simulink model "seEstimatingAssemblyLineThroughput"  (R2020b)
settings: Solver=VariableStepAuto  StartTime=0.0  StopTime=86407  FixedStep=7  RelTol=1e-3
PostLoadFcn:
  | excelFile   = [matlabroot...
  |   '/examples/simevents/data/seEstimatingAssemblyLineThroughput.xlsx'];
  | 
  | schedule    = xlsread(excelFile, 'MfgSchedule');      % Part Scheduling information
  | optimes     = xlsread(excelFile, 'OperationTimes');  % Operation Times
  | parameters  = xlsread(excelFile, 'Parameters');      % Simulation Parameters
  | 
  | numMfgWorkers = parameters(1); 		 % number of workers in Manufacturing area
  | numInspectWorkers = parameters(2); 	 % number of workers in Inspection area
  | discard_rate = parameters(4)/100; 	                     % quality rejection rate
  | seed = 12345;                     	                     % random number seed
  | requirements = xlsread(excelFile, 'Requirements');
  | scheduleID = 4;                                                        % The column number to read from excel
undefined symbols (not defined in the file or in its folder): m, n, openFastenGate, openInspect1Gate, openInspect2Gate, openInspect3Gate, openMilling1Gate, openMilling2Gate
libraries: sldelib x4, bonsai_library x1
CloseFcn:
  | clear discard_rate excelFile logsout numInspectWorkers numMfgWorkers optimes parameters requirements schedule scheduleID seed;
settings Model: Creator=The MathWorks, Inc.  LastModifiedBy=jomcdowe
settings DataIOCC: SaveOutput=off  SaveTime=off  ReturnWorkspaceOutputs=off
settings DebuggingCC: ArithmeticOperatorsInVariantConditions=warning
settings SFSimCC: SimUseLocalCustomCode=off  CustomCodeUndefinedFunction=UseInterfaceOnly
settings RTWCC: RTWUseLocalCustomCode=off
settings CodeAppCC: StateflowObjectComments=on

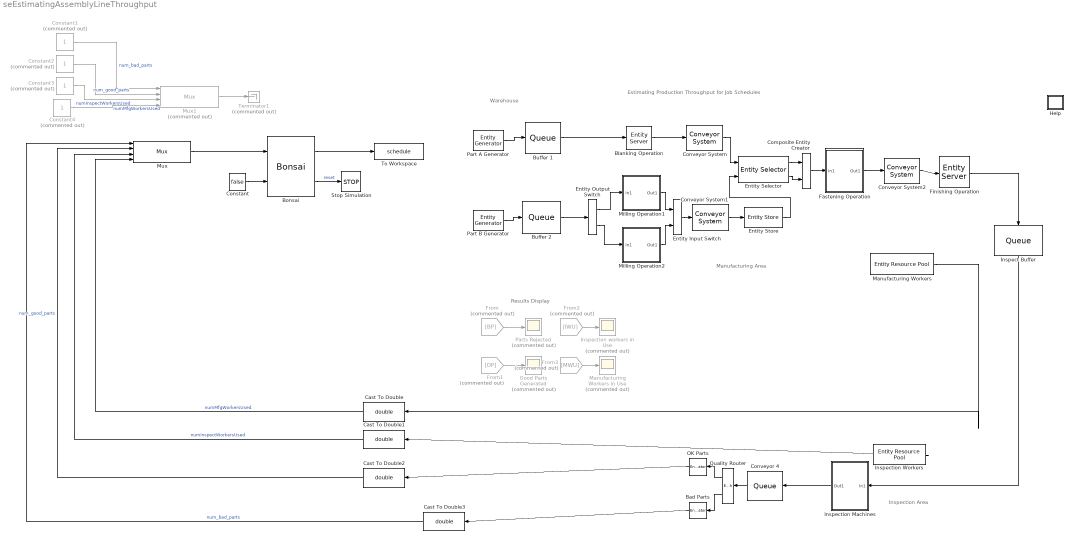
== system seEstimatingAssemblyLineThroughput ==
  note: Warehouse
  note: Results Display
  note: Manufacturing Area
  note: Estimating Production Throughput for Job Schedules
  note: Inspection Area
  Bad Parts : EntityTerminator  InputPortMessageModes=m  NumberEntitiesArrived=on
      settings: OutputPortMap=o0
  Blanking Operation : EntityServer  InputPortMessageModes=m  OutputPortMessageModes=m  Capacity=1  ServiceTimeSource=MATLAB action  ServiceTimeAction=|
      | % The times on the servers are going to vary
      | % as a normal dist, with std-dev of 'variation'.
      | 
      | persistent rngInit;
      | if isempty(rngInit)
      |     rng(seed);
      |     rngInit = true;
      | end
      | 
      | variation = parameters(5)/100;    % variation over nominal
      | nominalTime = optimes(entity.Variant, 2);
      | stdDev = nominalTime*variation;
      | 
      | % Pattern: Gaussian (normal) distribution
      | dt = nominalTime + stdDev * randn;
      mask Display: image([matlabroot,'/examples/simevents/data/SLDEBlanking.gif']);
  Bonsai : bonsai_library/Bonsai  sampleTime=[68400, 0]
      settings: SourceProductName=Bonsai Toolbox
  Buffer 1 : Queue  InputPortMessageModes=m  OutputPortMessageModes=m  Capacity=4
      mask Display: image([matlabroot,'/examples/simevents/data/SLDEPallet.png']);
  Buffer 2 : Queue  InputPortMessageModes=m  OutputPortMessageModes=m  Capacity=4
      mask Display: image([matlabroot,'/examples/simevents/data/SLDEPallet.png']);
  Cast To Double{,1..3} (4 alike) : DataTypeConversion  OutDataTypeStr=double
  Composite Entity Creator : CompositeEntityCreator  InputPortMessageModes=m,m  OutputPortMessageModes=m  EntityTypeName=Combined  InputEntityName=Part_A|Part_B
      settings: InputPortMap=u0,u1
  Constant : Constant  Value=false
  Constant{1..4} (4 alike) : Constant  Commented=on
  Conveyor 4 : Queue  InputPortMessageModes=m  OutputPortMessageModes=m  Capacity=2  EntryAction=|
      | % Set the percentage of parts
      | % that have to be discarded
      | % discard_rate = 0.05;
      | 
      | flip = rand();
      | if flip > discard_rate
      |     entity.Part_A.Rework = 1;    % rework not needed
      | else
      |     entity.Part_A.Rework = 2;    % rework needed
      | end
      mask Display: image([matlabroot,'/examples/simevents/data/SLDEFlatPallet.jpg']);
  Conveyor System : sldelib/Conveyor System  mConveyorLength=100  mConveyorSpeedSource=Dialog  mConveyorSpeed=20  mInitialConveyorSpeed=1000  mMinDisBetEntity=0  mEntityLengthSource=Dialog  mEntityLength=30  mEntityLengthAttrName=Length  mOutputBlockedOpt=Accumulate  mErrorUponFullOpt=off  mNumEntitiesDepOpt=off  mNumEntitiesInBlockOpt=off  mEntityPendingOpt=off  mNumExtractedFromBlockOpt=off  mConveyorSpeedOpt=off
      settings: SourceProductName=SimEvents
  Conveyor System1 : sldelib/Conveyor System  mConveyorLength=100  mConveyorSpeedSource=Dialog  mConveyorSpeed=20  mInitialConveyorSpeed=1000  mMinDisBetEntity=0  mEntityLengthSource=Dialog  mEntityLength=30  mEntityLengthAttrName=Length  mOutputBlockedOpt=Accumulate  mErrorUponFullOpt=off  mNumEntitiesDepOpt=off  mNumEntitiesInBlockOpt=off  mEntityPendingOpt=off  mNumExtractedFromBlockOpt=off  mConveyorSpeedOpt=off
      settings: SourceProductName=SimEvents
  Conveyor System2 : sldelib/Conveyor System  mConveyorLength=100  mConveyorSpeedSource=Dialog  mConveyorSpeed=20  mInitialConveyorSpeed=1000  mMinDisBetEntity=0  mEntityLengthSource=Dialog  mEntityLength=30  mEntityLengthAttrName=Length  mOutputBlockedOpt=Accumulate  mErrorUponFullOpt=off  mNumEntitiesDepOpt=off  mNumEntitiesInBlockOpt=off  mEntityPendingOpt=off  mNumExtractedFromBlockOpt=off  mConveyorSpeedOpt=off
      settings: SourceProductName=SimEvents
  Entity Input Switch : EntityInputSwitch  InputPortMessageModes=m,m  OutputPortMessageModes=m
  Entity Output Switch : EntityOutputSwitch  InputPortMessageModes=m  OutputPortMessageModes=m,m  SwitchAttributeName=Attribute1
  Entity Selector : sldelib/Entity Selector  mNumberOfStreams=1  mKeyEntityAttributeName='Variant'  mEntityAttributeName='VariantB'  mMatchingNumberSource=Dialog  mNumberOfMatches=1  mNumberOfMatchesAttribute=Name  mNumEntitiesDepOpt=off  mNumEntitiesInBlockOpt=off  mNumEntitiesExtractedOpt=off
      settings: SourceProductName=SimEvents
  Entity Store : EntityStore  InputPortMessageModes=m  OutputPortMessageModes=m  Capacity=4
      settings: OutputPortMap=o4
  Fastening Operation : Subsystem
      mask Display: image([matlabroot,'/examples/simevents/data/SLDEFasteningMachine.jpg']);
  Finishing Operation : EntityServer  InputPortMessageModes=m  OutputPortMessageModes=m  Capacity=1  ServiceTimeSource=MATLAB action  ServiceTimeAction=|
      | % The times on the servers are going to vary
      | % as a normal dist, with std-dev of 'variation'.
      | 
      | persistent rngInit;
      | if isempty(rngInit)
      |     rng(seed);
      |     rngInit = true;
      | end
      | 
      | variation = parameters(5)/100;    % variation over nominal
      | nominalTime = optimes(entity.Part_A.Variant, 6);
      | stdDev = nominalTime*variation;
      | 
      | % Pattern: Gaussian (normal) distribution
      | dt = nominalTime + stdDev * randn;
      mask Display: image([matlabroot,'/examples/simevents/data/SLDEFinishing.jpg']);
  From : From  Commented=on  GotoTag=BP
  From1 : From  Commented=on  GotoTag=OP
  From2 : From  Commented=on  GotoTag=IWU
  From3 : From  Commented=on  GotoTag=MWU
  Good Parts Generated : Scope  Commented=on
  Help : Subsystem
      settings: OpenFcn=showExample('simevents/EstimatingAssemblyLineThroughputExample');
      mask Display: disp('?')
  Inspect Buffer : Queue  InputPortMessageModes=m  OutputPortMessageModes=m  Capacity=4
      mask Display: image([matlabroot,'/examples/simevents/data/SLDEPallet.png']);
  Inspection Machines : Subsystem
      mask Display: image([matlabroot,'/examples/simevents/data/SLDEInspectMachine.png']);
  Inspection Workers : EntityResourcePool  ResourceName=InspectionWorkers  ResourceAmount=numInspectWorkers  AmountInUse=on
  Inspection workers in Use : Scope  Commented=on
  Manufacturing Workers : EntityResourcePool  ResourceName=MillingFasteningWorkers  ResourceAmount=numMfgWorkers  AmountInUse=on
  Manufacturing Workers in Use : Scope  Commented=on
  Milling Operation1 : Subsystem
      mask Display: image([matlabroot,'/examples/simevents/data/SLDEMillingMachine.jpg']);
  Milling Operation2 : Subsystem
      mask Display: image([matlabroot,'/examples/simevents/data/SLDEMillingMachine.jpg']);
  Mux : Mux
      settings: DisplayOption=signals
  Mux1 : Mux  Commented=on
      settings: DisplayOption=signals
  OK Parts : EntityTerminator  InputPortMessageModes=m  NumberEntitiesArrived=on
      settings: OutputPortMap=o0
  Part A Generator : EntityGenerator  OutputPortMessageModes=m  TimeSource=MATLAB action  IntergenerationTimeAction=|  GenerateAction=|  AttributeName=Rework|Variant  AttributeInitialValue=1|1  EntityType=Structured  EntityTypeName=Part_A
      | persistent idx;
      | if isempty(idx)
      |     idx = 1;
      | end
      | 
      | % Set the Inter Generation Time (IGT)
      | dt = schedule(idx, 1);
      | if idx < length(schedule(:, 1))
      |     idx = idx + 1;
      | else
      |     idx = 1;    % go back to first part
      | end
      | persistent idx;
      | if isempty(idx)
      |     idx = 1;
      | end
      | 
      | % Set the variant
      | entity.Variant = schedule(idx, scheduleID);
      | 
      | % Book-keeping work
      | if idx < length(schedule(:, 1))
      |     idx = idx + 1;
      | else
      |     idx = 1;    % go back to first part
      | end
  Part B Generator : EntityGenerator  OutputPortMessageModes=m  TimeSource=MATLAB action  IntergenerationTimeAction=|  GenerateAction=|  AttributeName=VariantB  EntityType=Structured  EntityTypeName=Part_B
      | persistent idx;
      | if isempty(idx)
      |     idx = 1;
      | end
      | 
      | % Set the Inter Generation Time (IGT)
      | dt = schedule(idx, 1);
      | if idx < length(schedule(:, 1))
      |     idx = idx + 1;
      | else
      |     idx = 1;    % go back to first part
      | end
      | persistent idx;
      | if isempty(idx)
      |     idx = 1;
      | end
      | 
      | % Set the variant
      | entity.VariantB = schedule(idx, scheduleID);
      | if idx < length(schedule(:, 1))
      |     idx = idx + 1;
      | else
      |     idx = 1;    % go back to first part
      | end
  Parts Rejected : Scope  Commented=on
  Quality Router : EntityOutputSwitch  InputPortMessageModes=m  OutputPortMessageModes=m,m  SwitchingCriterion=From attribute  SwitchAttributeName=entity.Part_A.Rework
  Stop Simulation : Stop
  Terminator1 : Terminator  Commented=on
  To Workspace : ToWorkspace  VariableName=schedule  SaveFormat=Timeseries  SampleTime=-1
  wires:
  Part A Generator/1 -> Buffer 1/1
  Buffer 1/1 -> Blanking Operation/1
  Conveyor System2/1 -> Finishing Operation/1
  Entity Output Switch/1 -> Milling Operation1/1(In1)
  Entity Output Switch/2 -> Milling Operation2/1(In1)
  Milling Operation1/1(Out1) -> Entity Input Switch/1
  Finishing Operation/1 -> Inspect Buffer/1
  Part B Generator/1 -> Buffer 2/1
  Buffer 2/1 -> Entity Output Switch/1
  Entity Input Switch/1 -> Conveyor System1/1
  Milling Operation2/1(Out1) -> Entity Input Switch/2
  Blanking Operation/1 -> Conveyor System/1
  Composite Entity Creator/1 -> Fastening Operation/1(In1)
  Fastening Operation/1(Out1) -> Conveyor System2/1
  Quality Router/1 -> OK Parts/1
  Quality Router/2 -> Bad Parts/1
  Conveyor 4/1 -> Quality Router/1
  Inspect Buffer/1 -> Inspection Machines/1(In1)
  Inspection Machines/1(Out1) -> Conveyor 4/1
  From/1 -> Parts Rejected/1
  From1/1 -> Good Parts Generated/1
  From2/1 -> Inspection workers in Use/1
  From3/1 -> Manufacturing Workers in Use/1
  Conveyor System1/1 -> Entity Store/1
  Entity Store/1 -> Entity Selector/2
  Conveyor System/1 -> Entity Selector/1
  Entity Selector/1 -> Composite Entity Creator/1
  Entity Selector/2 -> Composite Entity Creator/2
  Constant/1 -> Bonsai/2
  Bonsai/2 -> Stop Simulation/1  "reset"
  Bonsai/1 -> To Workspace/1
  Bad Parts/1 -> Cast To Double3/1
  OK Parts/1 -> Cast To Double2/1
  Inspection Workers/1 -> Cast To Double1/1
  Manufacturing Workers/1 -> Cast To Double/1
  Cast To Double/1 -> Mux/4  "numMfgWorkersUsed"
  Cast To Double1/1 -> Mux/3  "numInspectWorkersUsed"
  Cast To Double2/1 -> Mux/2  "num_good_parts"
  Cast To Double3/1 -> Mux/1  "num_bad_parts"
  Mux1/1 -> Terminator1/1
  Mux/1 -> Bonsai/1
  Constant1/1 -> Mux1/1  "num_bad_parts"
  Constant2/1 -> Mux1/2  "num_good_parts"
  Constant3/1 -> Mux1/3  "numInspectWorkersUsed"
  Constant4/1 -> Mux1/4  "numMfgWorkersUsed"

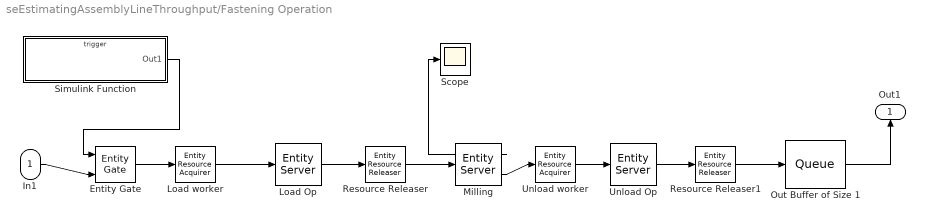
== system seEstimatingAssemblyLineThroughput/Fastening Operation ==
  In1 : Inport
  Entity Gate : EntityGate  InputPortMessageModes=m,m  OutputPortMessageModes=m  OperatingMode=Release gate  OpenGateAtSimulationStart=on
  Load Op : EntityServer  InputPortMessageModes=m  OutputPortMessageModes=m  Capacity=1  ServiceTimeValue=40
  Load worker : EntityResourceAcquirer  InputPortMessageModes=m  OutputPortMessageModes=m  ResourceName=MillingFasteningWorkers
      settings: OutputPortMap=o3
  Milling : EntityServer  InputPortMessageModes=m  OutputPortMessageModes=n,m  Capacity=1  ServiceTimeSource=MATLAB action  ServiceTimeAction=|  NumberEntitiesDeparted=on
      | % The times on the servers are going to vary
      | % as a normal dist, with std-dev of 'variation'.
      | 
      | persistent rngInit;
      | if isempty(rngInit)
      |     rng(seed);
      |     rngInit = true;
      | end
      | 
      | variation = parameters(5)/100;    % variation over nominal
      | nominalTime = optimes(entity.Part_A.Variant, 5);
      | stdDev = nominalTime*variation;
      | 
      | % Pattern: Gaussian (normal) distribution
      | dt = nominalTime + stdDev * randn;
      settings: OutputPortMap=o0,o9
      mask Display: image('SLDEFasteningMachine.jpg');
  Out Buffer of Size 1 : Queue  InputPortMessageModes=m  OutputPortMessageModes=m  Capacity=1  ExitAction=openFastenGate(1);
      mask Display: image('SLDEPallet.png');
  Resource Releaser : EntityResourceReleaser  InputPortMessageModes=m  OutputPortMessageModes=m
  Resource Releaser1 : EntityResourceReleaser  InputPortMessageModes=m  OutputPortMessageModes=m
  Scope : Scope
  Simulink Function : Subsystem  TreatAsAtomicUnit=on
  Unload Op : EntityServer  InputPortMessageModes=m  OutputPortMessageModes=m  Capacity=1  ServiceTimeValue=40
  Unload worker : EntityResourceAcquirer  InputPortMessageModes=m  OutputPortMessageModes=m  ResourceName=MillingFasteningWorkers
      settings: OutputPortMap=o3
  Out1 : Outport  VectorParamsAs1DForOutWhenUnconnected=off
  wires:
  Unload Op/1 -> Resource Releaser1/1
  Resource Releaser/1 -> Milling/1
  Load worker/1 -> Load Op/1
  Unload worker/1 -> Unload Op/1
  Milling/2 -> Unload worker/1
  Load Op/1 -> Resource Releaser/1
  In1/1 -> Entity Gate/2
  Entity Gate/1 -> Load worker/1
  Simulink Function/1(Out1) -> Entity Gate/1
  Resource Releaser1/1 -> Out Buffer of Size 1/1
  Out Buffer of Size 1/1 -> Out1/1
  Milling/1 -> Scope/1

== system seEstimatingAssemblyLineThroughput/Help ==

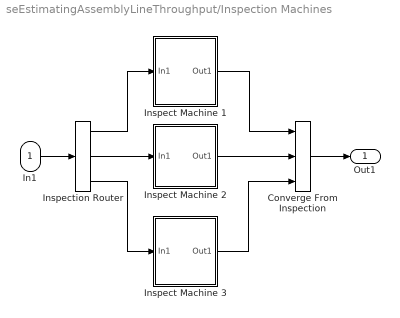
== system seEstimatingAssemblyLineThroughput/Inspection Machines ==
  In1 : Inport
  Converge From Inspection : EntityInputSwitch  InputPortMessageModes=m,m,m  OutputPortMessageModes=m  NumberInputPorts=3
      settings: InputPortMap=u1,u2,u3
  Inspect Machine 1 : Subsystem
      mask Display: image('SLDEInspectMachine.png');
  Inspect Machine 2 : Subsystem
      mask Display: image('SLDEInspectMachine.png');
  Inspect Machine 3 : Subsystem
      mask Display: image('SLDEInspectMachine.png');
  Inspection Router : EntityOutputSwitch  InputPortMessageModes=m  OutputPortMessageModes=m,m,m  NumberOutputPorts=3  SwitchAttributeName=Attribute1
      settings: OutputPortMap=o0,o1,o2
  Out1 : Outport  VectorParamsAs1DForOutWhenUnconnected=off
  wires:
  Converge From Inspection/1 -> Out1/1
  In1/1 -> Inspection Router/1
  Inspection Router/2 -> Inspect Machine 2/1(In1)
  Inspection Router/1 -> Inspect Machine 1/1(In1)
  Inspection Router/3 -> Inspect Machine 3/1(In1)
  Inspect Machine 1/1(Out1) -> Converge From Inspection/1
  Inspect Machine 2/1(Out1) -> Converge From Inspection/2
  Inspect Machine 3/1(Out1) -> Converge From Inspection/3

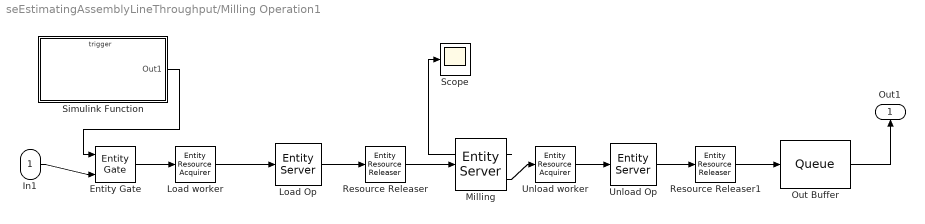
== system seEstimatingAssemblyLineThroughput/Milling Operation1 ==
  In1 : Inport
  Entity Gate : EntityGate  InputPortMessageModes=m,m  OutputPortMessageModes=m  OperatingMode=Release gate  OpenGateAtSimulationStart=on
  Load Op : EntityServer  InputPortMessageModes=m  OutputPortMessageModes=m  Capacity=1  ServiceTimeValue=40
  Load worker : EntityResourceAcquirer  InputPortMessageModes=m  OutputPortMessageModes=m  ResourceName=MillingFasteningWorkers
      settings: OutputPortMap=o3
  Milling : EntityServer  InputPortMessageModes=m  OutputPortMessageModes=n,m  Capacity=1  ServiceTimeSource=MATLAB action  ServiceTimeAction=|  NumberEntitiesDeparted=on
      | % The times on the servers are going to vary
      | % as a normal dist, with std-dev of 'variation'.
      | 
      | persistent rngInit;
      | if isempty(rngInit)
      |     rng(seed);
      |     rngInit = true;
      | end
      | 
      | variation = parameters(5)/100;    % variation over nominal
      | nominalTime = optimes(entity.VariantB, 3);
      | stdDev = nominalTime*variation;
      | 
      | % Pattern: Gaussian (normal) distribution
      | dt = nominalTime + stdDev * randn;
      settings: OutputPortMap=o0,o9
      mask Display: image('SLDEMillingMachine.jpg');
  Out Buffer : Queue  InputPortMessageModes=m  OutputPortMessageModes=m  Capacity=1  ExitAction=openMilling1Gate(1);
      mask Display: image('SLDEFlatPallet.jpg');
  Resource Releaser : EntityResourceReleaser  InputPortMessageModes=m  OutputPortMessageModes=m
  Resource Releaser1 : EntityResourceReleaser  InputPortMessageModes=m  OutputPortMessageModes=m
  Scope : Scope
  Simulink Function : Subsystem  TreatAsAtomicUnit=on
  Unload Op : EntityServer  InputPortMessageModes=m  OutputPortMessageModes=m  Capacity=1  ServiceTimeValue=40
  Unload worker : EntityResourceAcquirer  InputPortMessageModes=m  OutputPortMessageModes=m  ResourceName=MillingFasteningWorkers
      settings: OutputPortMap=o3
  Out1 : Outport  VectorParamsAs1DForOutWhenUnconnected=off
  wires:
  Unload Op/1 -> Resource Releaser1/1
  Resource Releaser/1 -> Milling/1
  Load worker/1 -> Load Op/1
  Unload worker/1 -> Unload Op/1
  Milling/2 -> Unload worker/1
  Load Op/1 -> Resource Releaser/1
  In1/1 -> Entity Gate/2
  Entity Gate/1 -> Load worker/1
  Simulink Function/1(Out1) -> Entity Gate/1
  Resource Releaser1/1 -> Out Buffer/1
  Out Buffer/1 -> Out1/1
  Milling/1 -> Scope/1

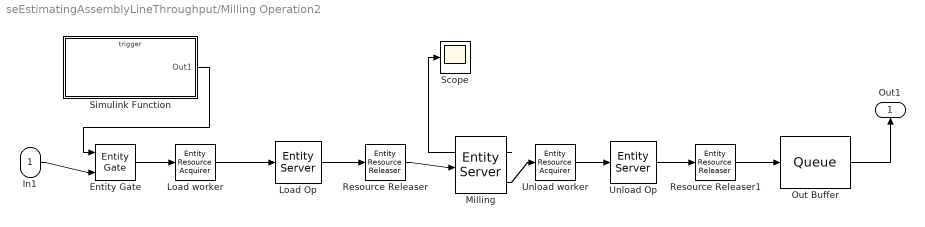
== system seEstimatingAssemblyLineThroughput/Milling Operation2 ==
  In1 : Inport
  Entity Gate : EntityGate  InputPortMessageModes=m,m  OutputPortMessageModes=m  OperatingMode=Release gate  OpenGateAtSimulationStart=on
  Load Op : EntityServer  InputPortMessageModes=m  OutputPortMessageModes=m  Capacity=1  ServiceTimeValue=40
  Load worker : EntityResourceAcquirer  InputPortMessageModes=m  OutputPortMessageModes=m  ResourceName=MillingFasteningWorkers
      settings: OutputPortMap=o3
  Milling : EntityServer  InputPortMessageModes=m  OutputPortMessageModes=n,m  Capacity=1  ServiceTimeSource=MATLAB action  ServiceTimeAction=|  NumberEntitiesDeparted=on
      | % The times on the servers are going to vary
      | % as a normal dist, with std-dev of 'variation'.
      | 
      | persistent rngInit;
      | if isempty(rngInit)
      |     rng(seed);
      |     rngInit = true;
      | end
      | 
      | variation = parameters(5)/100;    % variation over nominal
      | nominalTime = optimes(entity.VariantB, 4);
      | stdDev = nominalTime*variation;
      | 
      | % Pattern: Gaussian (normal) distribution
      | dt = nominalTime + stdDev * randn;
      settings: OutputPortMap=o0,o9
      mask Display: image('SLDEMillingMachine.jpg');
  Out Buffer : Queue  InputPortMessageModes=m  OutputPortMessageModes=m  Capacity=1  ExitAction=openMilling2Gate(1);
      mask Display: image('SLDEFlatPallet.jpg');
  Resource Releaser : EntityResourceReleaser  InputPortMessageModes=m  OutputPortMessageModes=m
  Resource Releaser1 : EntityResourceReleaser  InputPortMessageModes=m  OutputPortMessageModes=m
  Scope : Scope
  Simulink Function : Subsystem  TreatAsAtomicUnit=on
  Unload Op : EntityServer  InputPortMessageModes=m  OutputPortMessageModes=m  Capacity=1  ServiceTimeValue=40
  Unload worker : EntityResourceAcquirer  InputPortMessageModes=m  OutputPortMessageModes=m  ResourceName=MillingFasteningWorkers
      settings: OutputPortMap=o3
  Out1 : Outport  VectorParamsAs1DForOutWhenUnconnected=off
  wires:
  Milling/1 -> Scope/1
  Out Buffer/1 -> Out1/1
  Resource Releaser1/1 -> Out Buffer/1
  Simulink Function/1(Out1) -> Entity Gate/1
  Entity Gate/1 -> Load worker/1
  In1/1 -> Entity Gate/2
  Load Op/1 -> Resource Releaser/1
  Milling/2 -> Unload worker/1
  Unload worker/1 -> Unload Op/1
  Load worker/1 -> Load Op/1
  Resource Releaser/1 -> Milling/1
  Unload Op/1 -> Resource Releaser1/1

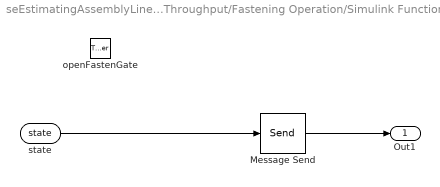
== system seEstimatingAssemblyLineThroughput/Fastening Operation/Simulink Function ==
  openFastenGate : TriggerPort  TriggerType=function-call  IsSimulinkFunction=on  FunctionName=openFastenGate  VariantControl=Variant
  Message Send : Send  OutputPortMessageModes=m
  state : ArgIn  DisableCoverage=on  ArgumentName=state
  Out1 : Outport  VectorParamsAs1DForOutWhenUnconnected=off
  wires:
  state/1 -> Message Send/1
  Message Send/1 -> Out1/1

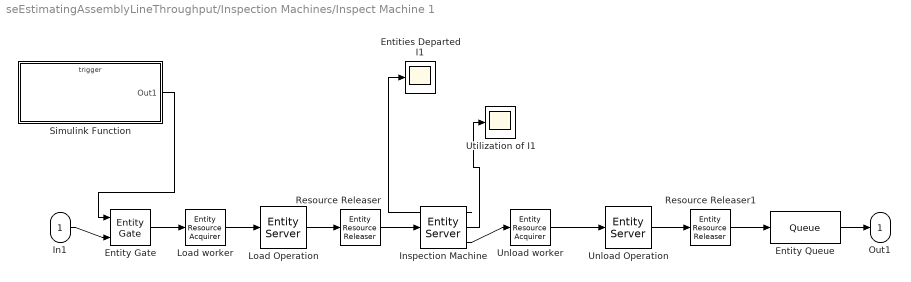
== system seEstimatingAssemblyLineThroughput/Inspection Machines/Inspect Machine 1 ==
  In1 : Inport
  Entities Departed I1 : Scope
  Entity Gate : EntityGate  InputPortMessageModes=m,m  OutputPortMessageModes=m  OperatingMode=Release gate  OpenGateAtSimulationStart=on
  Entity Queue : Queue  InputPortMessageModes=m  OutputPortMessageModes=m  Capacity=1  ExitAction=openInspect1Gate(1);
  Inspection Machine : EntityServer  InputPortMessageModes=m  OutputPortMessageModes=n,n,m  Capacity=1  ServiceTimeSource=MATLAB action  ServiceTimeAction=|  NumberEntitiesDeparted=on  Utilization=on
      | % The times on the servers are going to vary
      | % as a normal dist, with std-dev of 'variation'.
      | 
      | persistent rngInit;
      | if isempty(rngInit)
      |     rng(seed);
      |     rngInit = true;
      | end
      | 
      | variation = parameters(5)/100;    % variation over nominal
      | nominalTime = optimes(entity.Part_A.Variant, 7);
      | stdDev = nominalTime*variation;
      | 
      | % Pattern: Gaussian (normal) distribution
      | dt = nominalTime + stdDev * randn;
      settings: OutputPortMap=o0,o5,o9
  Load Operation : EntityServer  InputPortMessageModes=m  OutputPortMessageModes=m  Capacity=1  ServiceTimeValue=80
  Load worker : EntityResourceAcquirer  InputPortMessageModes=m  OutputPortMessageModes=m  ResourceName=InspectionWorkers
      settings: OutputPortMap=o3
  Resource Releaser : EntityResourceReleaser  InputPortMessageModes=m  OutputPortMessageModes=m
  Resource Releaser1 : EntityResourceReleaser  InputPortMessageModes=m  OutputPortMessageModes=m
  Simulink Function : Subsystem  TreatAsAtomicUnit=on
  Unload Operation : EntityServer  InputPortMessageModes=m  OutputPortMessageModes=m  Capacity=1  ServiceTimeValue=80
  Unload worker : EntityResourceAcquirer  InputPortMessageModes=m  OutputPortMessageModes=m  ResourceName=InspectionWorkers
      settings: OutputPortMap=o3
  Utilization of I1 : Scope
  Out1 : Outport  VectorParamsAs1DForOutWhenUnconnected=off
  wires:
  Unload Operation/1 -> Resource Releaser1/1
  Resource Releaser/1 -> Inspection Machine/1
  Load worker/1 -> Load Operation/1
  Unload worker/1 -> Unload Operation/1
  Inspection Machine/3 -> Unload worker/1
  Load Operation/1 -> Resource Releaser/1
  Inspection Machine/1 -> Entities Departed I1/1
  In1/1 -> Entity Gate/2
  Entity Gate/1 -> Load worker/1
  Simulink Function/1(Out1) -> Entity Gate/1
  Inspection Machine/2 -> Utilization of I1/1
  Resource Releaser1/1 -> Entity Queue/1
  Entity Queue/1 -> Out1/1

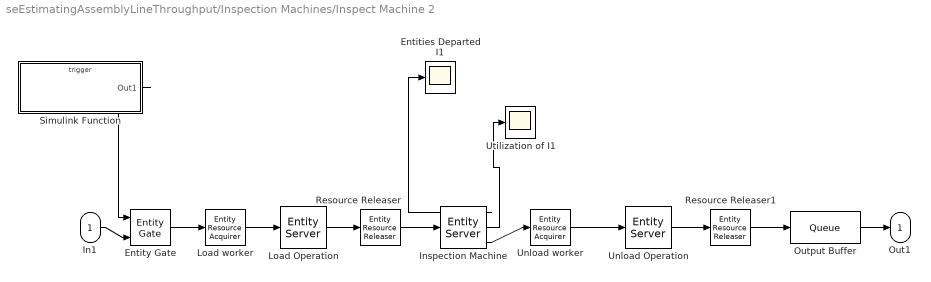
== system seEstimatingAssemblyLineThroughput/Inspection Machines/Inspect Machine 2 ==
  In1 : Inport
  Entities Departed I1 : Scope
  Entity Gate : EntityGate  InputPortMessageModes=m,m  OutputPortMessageModes=m  OperatingMode=Release gate  OpenGateAtSimulationStart=on
  Inspection Machine : EntityServer  InputPortMessageModes=m  OutputPortMessageModes=n,n,m  Capacity=1  ServiceTimeSource=MATLAB action  ServiceTimeAction=|  NumberEntitiesDeparted=on  Utilization=on
      | % The times on the servers are going to vary
      | % as a normal dist, with std-dev of 'variation'.
      | 
      | persistent rngInit;
      | if isempty(rngInit)
      |     rng(seed);
      |     rngInit = true;
      | end
      | 
      | variation = parameters(5)/100;    % variation over nominal
      | nominalTime = optimes(entity.Part_A.Variant, 8);
      | stdDev = nominalTime*variation;
      | 
      | % Pattern: Gaussian (normal) distribution
      | dt = nominalTime + stdDev * randn;
      settings: OutputPortMap=o0,o5,o9
  Load Operation : EntityServer  InputPortMessageModes=m  OutputPortMessageModes=m  Capacity=1  ServiceTimeValue=80
  Load worker : EntityResourceAcquirer  InputPortMessageModes=m  OutputPortMessageModes=m  ResourceName=InspectionWorkers
      settings: OutputPortMap=o3
  Output Buffer : Queue  InputPortMessageModes=m  OutputPortMessageModes=m  Capacity=1  ExitAction=openInspect2Gate(1);
  Resource Releaser : EntityResourceReleaser  InputPortMessageModes=m  OutputPortMessageModes=m
  Resource Releaser1 : EntityResourceReleaser  InputPortMessageModes=m  OutputPortMessageModes=m
  Simulink Function : Subsystem  TreatAsAtomicUnit=on
  Unload Operation : EntityServer  InputPortMessageModes=m  OutputPortMessageModes=m  Capacity=1  ServiceTimeValue=80
  Unload worker : EntityResourceAcquirer  InputPortMessageModes=m  OutputPortMessageModes=m  ResourceName=InspectionWorkers
      settings: OutputPortMap=o3
  Utilization of I1 : Scope
  Out1 : Outport  VectorParamsAs1DForOutWhenUnconnected=off
  wires:
  Output Buffer/1 -> Out1/1
  Resource Releaser1/1 -> Output Buffer/1
  Inspection Machine/2 -> Utilization of I1/1
  Simulink Function/1(Out1) -> Entity Gate/1
  Entity Gate/1 -> Load worker/1
  In1/1 -> Entity Gate/2
  Inspection Machine/1 -> Entities Departed I1/1
  Load Operation/1 -> Resource Releaser/1
  Inspection Machine/3 -> Unload worker/1
  Unload worker/1 -> Unload Operation/1
  Load worker/1 -> Load Operation/1
  Resource Releaser/1 -> Inspection Machine/1
  Unload Operation/1 -> Resource Releaser1/1

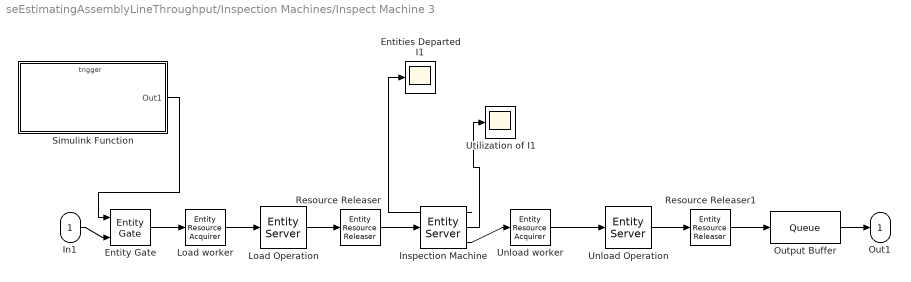
== system seEstimatingAssemblyLineThroughput/Inspection Machines/Inspect Machine 3 ==
  In1 : Inport
  Entities Departed I1 : Scope
  Entity Gate : EntityGate  InputPortMessageModes=m,m  OutputPortMessageModes=m  OperatingMode=Release gate  OpenGateAtSimulationStart=on
  Inspection Machine : EntityServer  InputPortMessageModes=m  OutputPortMessageModes=n,n,m  Capacity=1  ServiceTimeSource=MATLAB action  ServiceTimeAction=|  NumberEntitiesDeparted=on  Utilization=on
      | % The times on the servers are going to vary
      | % as a normal dist, with std-dev of 'variation'.
      | 
      | persistent rngInit;
      | if isempty(rngInit)
      |     rng(seed);
      |     rngInit = true;
      | end
      | 
      | variation = parameters(5)/100;    % variation over nominal
      | nominalTime = optimes(entity.Part_A.Variant, 9);
      | stdDev = nominalTime*variation;
      | 
      | % Pattern: Gaussian (normal) distribution
      | dt = nominalTime + stdDev * randn;
      settings: OutputPortMap=o0,o5,o9
  Load Operation : EntityServer  InputPortMessageModes=m  OutputPortMessageModes=m  Capacity=1  ServiceTimeValue=80
  Load worker : EntityResourceAcquirer  InputPortMessageModes=m  OutputPortMessageModes=m  ResourceName=InspectionWorkers
      settings: OutputPortMap=o3
  Output Buffer : Queue  InputPortMessageModes=m  OutputPortMessageModes=m  Capacity=1  ExitAction=openInspect3Gate(1);
  Resource Releaser : EntityResourceReleaser  InputPortMessageModes=m  OutputPortMessageModes=m
  Resource Releaser1 : EntityResourceReleaser  InputPortMessageModes=m  OutputPortMessageModes=m
  Simulink Function : Subsystem  TreatAsAtomicUnit=on
  Unload Operation : EntityServer  InputPortMessageModes=m  OutputPortMessageModes=m  Capacity=1  ServiceTimeValue=80
  Unload worker : EntityResourceAcquirer  InputPortMessageModes=m  OutputPortMessageModes=m  ResourceName=InspectionWorkers
      settings: OutputPortMap=o3
  Utilization of I1 : Scope
  Out1 : Outport  VectorParamsAs1DForOutWhenUnconnected=off
  wires:
  Unload Operation/1 -> Resource Releaser1/1
  Resource Releaser/1 -> Inspection Machine/1
  Load worker/1 -> Load Operation/1
  Unload worker/1 -> Unload Operation/1
  Inspection Machine/3 -> Unload worker/1
  Load Operation/1 -> Resource Releaser/1
  Inspection Machine/1 -> Entities Departed I1/1
  In1/1 -> Entity Gate/2
  Entity Gate/1 -> Load worker/1
  Simulink Function/1(Out1) -> Entity Gate/1
  Inspection Machine/2 -> Utilization of I1/1
  Resource Releaser1/1 -> Output Buffer/1
  Output Buffer/1 -> Out1/1

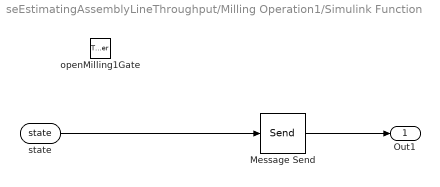
== system seEstimatingAssemblyLineThroughput/Milling Operation1/Simulink Function ==
  openMilling1Gate : TriggerPort  TriggerType=function-call  IsSimulinkFunction=on  FunctionName=openMilling1Gate  VariantControl=Variant
  Message Send : Send  OutputPortMessageModes=m
  state : ArgIn  DisableCoverage=on  ArgumentName=state
  Out1 : Outport  VectorParamsAs1DForOutWhenUnconnected=off
  wires:
  state/1 -> Message Send/1
  Message Send/1 -> Out1/1

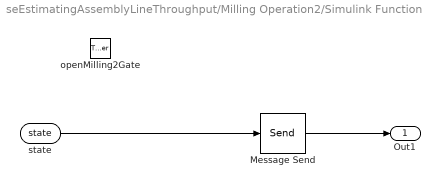
== system seEstimatingAssemblyLineThroughput/Milling Operation2/Simulink Function ==
  openMilling2Gate : TriggerPort  TriggerType=function-call  IsSimulinkFunction=on  FunctionName=openMilling2Gate  VariantControl=Variant
  Message Send : Send  OutputPortMessageModes=m
  state : ArgIn  DisableCoverage=on  ArgumentName=state
  Out1 : Outport  VectorParamsAs1DForOutWhenUnconnected=off
  wires:
  Message Send/1 -> Out1/1
  state/1 -> Message Send/1

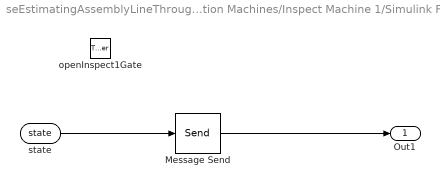
== system seEstimatingAssemblyLineThroughput/Inspection Machines/Inspect Machine 1/Simulink Function ==
  openInspect1Gate : TriggerPort  TriggerType=function-call  IsSimulinkFunction=on  FunctionName=openInspect1Gate  VariantControl=Variant
  Message Send : Send  OutputPortMessageModes=m
  state : ArgIn  DisableCoverage=on  ArgumentName=state
  Out1 : Outport  VectorParamsAs1DForOutWhenUnconnected=off
  wires:
  state/1 -> Message Send/1
  Message Send/1 -> Out1/1

== system seEstimatingAssemblyLineThroughput/Inspection Machines/Inspect Machine 2/Simulink Function ==
  openInspect2Gate : TriggerPort  TriggerType=function-call  IsSimulinkFunction=on  FunctionName=openInspect2Gate  VariantControl=Variant
  Message Send : Send  OutputPortMessageModes=m
  state : ArgIn  DisableCoverage=on  ArgumentName=state
  Out1 : Outport  VectorParamsAs1DForOutWhenUnconnected=off
  wires:
  Message Send/1 -> Out1/1
  state/1 -> Message Send/1

== system seEstimatingAssemblyLineThroughput/Inspection Machines/Inspect Machine 3/Simulink Function ==
  openInspect3Gate : TriggerPort  TriggerType=function-call  IsSimulinkFunction=on  FunctionName=openInspect3Gate  VariantControl=Variant
  Message Send : Send  OutputPortMessageModes=m
  state : ArgIn  DisableCoverage=on  ArgumentName=state
  Out1 : Outport  VectorParamsAs1DForOutWhenUnconnected=off
  wires:
  state/1 -> Message Send/1
  Message Send/1 -> Out1/1
